simulink library "Lib_Piccolo"  (R2018b)
settings: Solver=VariableStepAuto  StartTime=0.0  StopTime=10.0  RelTol=1e-3
values from neighbouring files (symbols this model uses):
  AccelErrInt2Brakes = 0.15    [SimulationControlConfig16P.m]    (also in SimulationControlConfig16P_F0.m; SimulationControlConfig16P_F2.m; SimulationControlConfig16P_LEGACY.m; SimulationControlConfigTAILLESS.m = 0.2)
  AileronMax = 25    [SimulationControlConfig16P.m]    (also in SimulationControlConfig16P_F0.m; SimulationControlConfig16P_F2.m; SimulationControlConfig16P_LEGACY.m; SimulationControlConfigTAILLESS.m)
  AileronPower = 0.00268    [SimulationControlConfig16P.m]    (also in SimulationControlConfig16P_F0.m; SimulationControlConfig16P_F2.m; SimulationControlConfig16P_LEGACY.m; SimulationControlConfigTAILLESS.m = 0.002266)
  AileronSurfaceMax = 45    [SimulationControlConfig16P.m]    (also in SimulationControlConfig16P_F0.m; SimulationControlConfig16P_F2.m; SimulationControlConfig16P_LEGACY.m; SimulationControlConfigTAILLESS_CGAFT_F0.m = 25)
  AileronTrim = 0    [SimulationControlConfig16P.m]    (also in SimulationControlConfig16P_F0.m; SimulationControlConfig16P_F2.m; SimulationControlConfig16P_LEGACY.m; SimulationControlConfigTAILLESS.m)
  Alt = 1000 + TerrainHeight    [SimulationStateConfig.m]
  AltCruise_m = Alt * 0.3048    [SimulationControlConfig16P.m]    (also in SimulationControlConfig16P_F2.m; SimulationControlConfigTAILLESS.m = Alt/3.28084; SimulationControlConfigTAILLESS_CGAFT_F0.m = 640; SimulationControlConfigTAILLESS_CGFWD_F0.m = 640)
  AltitudeRate2PitchCmdIntegratorInit = 0.1    [SimulationControlPre.m]
  AltMax = 10000    [SimulationControlConfig16P.m]    (also in SimulationControlConfig16P_F0.m; SimulationControlConfig16P_F2.m; SimulationControlConfig16P_LEGACY.m; SimulationControlConfigTAILLESS.m)
  AltMaxAccel = 2.5    [SimulationControlConfig16P.m]    (also in SimulationControlConfig16P_F0.m = 2; SimulationControlConfig16P_F2.m = 2; SimulationControlConfig16P_LEGACY.m = 0.9; SimulationControlConfigTAILLESS.m = 2)
  AltMin = 0    [SimulationControlConfig16P.m]    (also in SimulationControlConfig16P_F0.m; SimulationControlConfig16P_F2.m; SimulationControlConfig16P_LEGACY.m; SimulationControlConfigTAILLESS.m)
  AltRateCmd2Pitch = 0.26    [SimulationControlConfig16P.m]    (also in SimulationControlConfig16P_F0.m = 0.35; SimulationControlConfig16P_F2.m = 0.35; SimulationControlConfig16P_LEGACY.m = 0.6; SimulationControlConfigTAILLESS.m = 0.9)
  AltRateError2Pitch = 0.34    [SimulationControlConfig16P.m]    (also in SimulationControlConfig16P_F0.m = 0.61; SimulationControlConfig16P_F2.m = 0.61; SimulationControlConfig16P_LEGACY.m = 0.4; SimulationControlConfigTAILLESS.m = 0.3)
  AltRateErrorInt2Pitch = 0.61    [SimulationControlConfig16P.m]    (also in SimulationControlConfig16P_F0.m = 0.28; SimulationControlConfig16P_F2.m = 0.28; SimulationControlConfig16P_LEGACY.m = 0.45; SimulationControlConfigTAILLESS.m = 0.15)
  AltRateLpfCutOff = 3    [SimulationControlConfig16P.m]    (also in SimulationControlConfig16P_F0.m; SimulationControlConfig16P_F2.m; SimulationControlConfig16P_LEGACY.m; SimulationControlConfigTAILLESS.m = 5)
  AutoNosegear2Rudder = 26    [SimulationControlConfig16P.m]    (also in SimulationControlConfig16P_F0.m; SimulationControlConfig16P_F2.m; SimulationControlConfig16P_LEGACY.m; SimulationControlConfigTAILLESS.m = 25.2)
  b = 5.54    [SimulationControlConfig16P.m]    (also in SimulationControlConfig16P_F0.m; SimulationControlConfig16P_F2.m; SimulationControlConfig16P_LEGACY.m; SimulationControlConfigTAILLESS.m = 2.37)
  Bank2AileronIntegratorInit = 0    [SimulationControlPre.m]
  BankMax_User = BankMax_User/180*pi    (= 0.610865238198)    [SimulationControlConfig16P.m]    (also in SimulationControlConfig16P_F0.m = 0.523598775598; SimulationControlConfig16P_F2.m = 0.523598775598; SimulationControlConfig16P_LEGACY.m = 0.523598775598; SimulationControlConfigTAILLESS.m = 0.558505360638)
  baseLegFlaps = 20    [SimulationControlConfig16P.m]    (also in SimulationControlConfig16P_F0.m; SimulationControlConfig16P_F2.m = 15; SimulationControlConfig16P_LEGACY.m = 0; SimulationControlConfigTAILLESS.m = 0)
  C = GeneticOpt.C    [SimulationCostFunction.m]
  c = Sw/b    (= 0.841696750903)    [SimulationControlConfig16P.m]    (also in SimulationControlConfig16P_F0.m; SimulationControlConfig16P_F2.m; SimulationControlConfig16P_LEGACY.m; SimulationControlConfigTAILLESS.m = 0.354008438819)
  cell2WheelFactorMG = 5.98    [SimulationSensorConfig16P_LEGACY.m]
  cell2WheelFactorNG = 1    [SimulationSensorConfig16P_LEGACY.m]
  cellSatMaxMG = 15000    [SimulationSensorConfig16P.m]    (also in SimulationSensorConfig16P_LEGACY.m; SimulationSensorConfigTAILLESS7P.m; SimulationSensorConfigUTAIL7P.m)
  cellSatMaxNG = 1000    [SimulationSensorConfig16P.m]    (also in SimulationSensorConfig16P_LEGACY.m; SimulationSensorConfigTAILLESS7P.m; SimulationSensorConfigUTAIL7P.m)
  cellSatMinMG = -15000    [SimulationSensorConfig16P.m]    (also in SimulationSensorConfig16P_LEGACY.m; SimulationSensorConfigTAILLESS7P.m; SimulationSensorConfigUTAIL7P.m)
  cellSatMinNG = -1000    [SimulationSensorConfig16P.m]    (also in SimulationSensorConfig16P_LEGACY.m; SimulationSensorConfigTAILLESS7P.m; SimulationSensorConfigUTAIL7P.m)
  CL_Limit = CL_Max    (= 0.54)    [SimulationControlConfig16P.m]    (also in SimulationControlConfig16P_F0.m; SimulationControlConfig16P_F2.m = 0.638; SimulationControlConfig16P_LEGACY.m; SimulationControlConfigTAILLESS.m = 0.525)
  CL_Max = 0.54    [SimulationControlConfig16P.m]    (also in SimulationControlConfig16P_F0.m; SimulationControlConfig16P_F2.m = 0.638; SimulationControlConfig16P_LEGACY.m; SimulationControlConfigTAILLESS.m = 0.525)
  CL_Max_Nom = 0.465    [SimulationControlConfig16P.m]    (also in SimulationControlConfig16P_F0.m; SimulationControlConfig16P_F2.m = 0.563; SimulationControlConfig16P_LEGACY.m; SimulationControlConfigTAILLESS.m = 0.39)
  CL_Min = 0    [SimulationControlConfig16P.m]    (also in SimulationControlConfig16P_F0.m; SimulationControlConfig16P_F2.m; SimulationControlConfig16P_LEGACY.m; SimulationControlConfigTAILLESS.m)
  ClimbMaxFraction = 0.35    [SimulationControlConfig16P.m]    (also in SimulationControlConfig16P_F0.m = 0.17; SimulationControlConfig16P_F2.m = 0.17; SimulationControlConfig16P_LEGACY.m = 0.24; SimulationControlConfigTAILLESS.m = 0.21)
  ClimboutMaxBank = 7.0    (= 7)    [SimulationControlConfig16P.m]    (also in SimulationControlConfig16P_F0.m; SimulationControlConfig16P_F2.m; SimulationControlConfig16P_LEGACY.m; SimulationControlConfigTAILLESS.m = 5)
  ClimboutTimer = 7.0    (= 7)    [SimulationControlConfig16P.m]    (also in SimulationControlConfig16P_F0.m; SimulationControlConfig16P_F2.m; SimulationControlConfig16P_LEGACY.m; SimulationControlConfigTAILLESS.m)
  dCl_per_dFlap = 0.005581818    [SimulationControlConfig16P.m]    (also in SimulationControlConfig16P_F0.m = 0; SimulationControlConfig16P_F2.m = 0.0065; SimulationControlConfig16P_LEGACY.m = 0; SimulationControlConfigTAILLESS.m = 0)
  DecelerationCmd = 3.1    [SimulationControlConfig16P.m]    (also in SimulationControlConfig16P_F0.m; SimulationControlConfig16P_F2.m; SimulationControlConfig16P_LEGACY.m; SimulationControlConfigTAILLESS.m = 0.1)
  DeRotateLogicEndTimer = abs((NoseDownLimit_Deg-1)/DeRotateRamp_Dps)    [SimulationControlConfig16P.m]    (also in SimulationControlConfig16P_F0.m; SimulationControlConfig16P_F2.m; SimulationControlConfig16P_LEGACY.m; SimulationControlConfigTAILLESS.m)
  DeRotateLogicHoldNoseUpTimer = 0.1    [SimulationControlConfig16P.m]    (also in SimulationControlConfig16P_F0.m; SimulationControlConfig16P_F2.m; SimulationControlConfig16P_LEGACY.m; SimulationControlConfigTAILLESS.m)
  DeRotateLogicTimerTimeout = 2    [SimulationControlConfig16P.m]    (also in SimulationControlConfig16P_F0.m; SimulationControlConfig16P_F2.m; SimulationControlConfig16P_LEGACY.m; SimulationControlConfigTAILLESS.m)
  DeRotateLowerCmdSaturation = 0    [SimulationControlConfig16P.m]    (also in SimulationControlConfig16P_F0.m; SimulationControlConfig16P_F2.m; SimulationControlConfig16P_LEGACY.m; SimulationControlConfigTAILLESS.m)
  DeRotateRamp_Dps = 3    [SimulationControlConfig16P.m]    (also in SimulationControlConfig16P_F0.m; SimulationControlConfig16P_F2.m; SimulationControlConfig16P_LEGACY.m; SimulationControlConfigTAILLESS.m = 8)
  DeRotateUpperCmdSaturation = 7    [SimulationControlConfig16P.m]    (also in SimulationControlConfig16P_F0.m; SimulationControlConfig16P_F2.m; SimulationControlConfig16P_LEGACY.m; SimulationControlConfigTAILLESS.m)
  DescentMaxFraction = 0.22    [SimulationControlConfig16P.m]    (also in SimulationControlConfig16P_F0.m = 0.2; SimulationControlConfig16P_F2.m = 0.2; SimulationControlConfig16P_LEGACY.m = 0.2; SimulationControlConfigTAILLESS.m = 0.17)
  DesktopSimTerrainOffset_m = 0.406    [SimulationAircraftConfig.m]
  downwindFlaps = 0    [SimulationControlConfig16P.m]    (also in SimulationControlConfig16P_F0.m; SimulationControlConfig16P_F2.m = 15; SimulationControlConfig16P_LEGACY.m; SimulationControlConfigTAILLESS.m)
  downwindSplitAil = 0    [SimulationControlConfig16P_F2.m]
  DP_init = 0.5*1.225*V_init^2    [SimulationControlConfig16P.m]    (also in SimulationControlConfig16P_F0.m; SimulationControlConfig16P_F2.m; SimulationControlConfig16P_LEGACY.m; SimulationControlConfigTAILLESS.m)
  dscNoiseMG = 1    [SimulationSensorConfig16P_LEGACY.m]
  dscNoiseNG = 0.25    [SimulationSensorConfig16P_LEGACY.m]
  DSCnumBits = 24    [SimulationSensorConfig16P.m]    (also in SimulationSensorConfig16P_LEGACY.m; SimulationSensorConfigTAILLESS7P.m; SimulationSensorConfigUTAIL7P.m)
  DSCRangeMaxMG = 15000    [SimulationSensorConfig16P.m]    (also in SimulationSensorConfig16P_LEGACY.m; SimulationSensorConfigTAILLESS7P.m; SimulationSensorConfigUTAIL7P.m)
  DSCRangeMaxNG = 1000    [SimulationSensorConfig16P.m]    (also in SimulationSensorConfig16P_LEGACY.m; SimulationSensorConfigTAILLESS7P.m; SimulationSensorConfigUTAIL7P.m)
  DSCRangeMinMG = -15000    [SimulationSensorConfig16P.m]    (also in SimulationSensorConfig16P_LEGACY.m; SimulationSensorConfigTAILLESS7P.m; SimulationSensorConfigUTAIL7P.m)
  DSCRangeMinNG = -1000    [SimulationSensorConfig16P.m]    (also in SimulationSensorConfig16P_LEGACY.m; SimulationSensorConfigTAILLESS7P.m; SimulationSensorConfigUTAIL7P.m)
  dt = DLLSim.dt    [SimulationTimeStep.m]    (also in SimulationTrim.m = 0.02)
  EarlyTouchdownThreshold = 3.0    (= 3)    [SimulationControlConfig16P.m]    (also in SimulationControlConfig16P_F0.m; SimulationControlConfig16P_F2.m; SimulationControlConfig16P_LEGACY.m; SimulationControlConfigTAILLESS.m)
  ElevatorDeflectionRate = 15    [SimulationControlConfig16P.m]    (also in SimulationControlConfig16P_F0.m; SimulationControlConfig16P_F2.m; SimulationControlConfig16P_LEGACY.m = 12; SimulationControlConfigTAILLESS.m = 5)
  ElevatorMax = 25    [SimulationControlConfig16P.m]    (also in SimulationControlConfig16P_F0.m; SimulationControlConfig16P_F2.m; SimulationControlConfig16P_LEGACY.m; SimulationControlConfigTAILLESS.m)
  ElevatorPower = -0.002209    [SimulationControlConfig16P.m]    (also in SimulationControlConfig16P_F0.m; SimulationControlConfig16P_F2.m; SimulationControlConfig16P_LEGACY.m; SimulationControlConfigTAILLESS.m = -0.002668)
  ElevatorTrim = -3.5    [SimulationControlConfig16P.m]    (also in SimulationControlConfig16P_F0.m; SimulationControlConfig16P_F2.m; SimulationControlConfig16P_LEGACY.m; SimulationControlConfigTAILLESS.m = -3)
  elevonBias = 0    [SimulationControlConfig16P.m]    (also in SimulationControlConfig16P_F0.m; SimulationControlConfig16P_F2.m; SimulationControlConfig16P_LEGACY.m; SimulationControlConfigTAILLESS.m)
  Enable_TAS_Protection = 0    [SimulationControlConfig16P.m]    (also in SimulationControlConfig16P_F0.m; SimulationControlConfig16P_F2.m; SimulationControlConfig16P_LEGACY.m; SimulationControlConfigTAILLESS.m)
  EnableCrossTrackAbort = 1    [SimulationControlConfig16P.m]    (also in SimulationControlConfigTAILLESS.m; SimulationControlConfigTAILLESS_CGAFT_F0.m; SimulationControlConfigTAILLESS_CGFWD_F0.m; SimulationControlConfigTAILLESS_CGFWD_F2.m)
  EnergyBandwidth = 0.04    [SimulationControlConfig16P.m]    (also in SimulationControlConfig16P_F0.m = 0.03; SimulationControlConfig16P_F2.m = 0.03; SimulationControlConfig16P_LEGACY.m = 0.02; SimulationControlConfigTAILLESS.m = 0.06)
  EngineLhFuelCut = 0    [SimulationAircraftConfig.m]
  EngineRhFuelCut = 0    [SimulationAircraftConfig.m]
  FastThrottleRate = 0.075    [SimulationControlConfig16P.m]    (also in SimulationControlConfig16P_F0.m = 0.05; SimulationControlConfig16P_F2.m = 0.05; SimulationControlConfig16P_LEGACY.m = 0.05; SimulationControlConfigTAILLESS.m = 0.1)
  FilterWarmUpTime = 2    [SimulationSensorConfig16P.m]    (also in SimulationSensorConfig16P_LEGACY.m; SimulationSensorConfigTAILLESS7P.m; SimulationSensorConfigUTAIL7P.m)
  finalApproachFlaps = 20    [SimulationControlConfig16P.m]    (also in SimulationControlConfig16P_F0.m; SimulationControlConfig16P_F2.m = 15; SimulationControlConfig16P_LEGACY.m = 0; SimulationControlConfigTAILLESS.m = 0)
  finalApproachSplitAil = 20    [SimulationControlConfig16P_F2.m]
  FinalDescentSlope_Deg = testPlans(testIndx).descentSlope    [SimulationControlConfig16P.m]    (also in SimulationControlConfig16P_F0.m; SimulationControlConfig16P_F2.m; SimulationControlConfig16P_LEGACY.m; SimulationControlConfigTAILLESS.m)
  flapMax = 0    [SimulationControlConfig16P.m]    (also in SimulationControlConfig16P_F0.m = 35; SimulationControlConfig16P_F2.m = 33; SimulationControlConfig16P_LEGACY.m; SimulationControlConfigTAILLESS.m)
  flapRate = 7.5    [SimulationControlConfig16P.m]    (also in SimulationControlConfig16P_F0.m; SimulationControlConfig16P_F2.m; SimulationControlConfig16P_LEGACY.m; SimulationControlConfigTAILLESS.m = 6.6)
  FlareHeight = 5    [SimulationControlConfig16P.m]    (also in SimulationControlConfig16P_F0.m; SimulationControlConfig16P_F2.m; SimulationControlConfig16P_LEGACY.m = 4.8; SimulationControlConfigTAILLESS.m = 2.75)
  FlareVerticalRate_mps = -0.4    [SimulationControlConfig16P.m]    (also in SimulationControlConfig16P_F0.m; SimulationControlConfig16P_F2.m; SimulationControlConfig16P_LEGACY.m = -0.5; SimulationControlConfigTAILLESS.m = -0.15)
  Fp_Aileron = 0.55*2*pi*RollRateLpfCutoff*dt    [SimulationControlConfig16P.m]    (also in SimulationControlConfig16P_F0.m; SimulationControlConfig16P_F2.m; SimulationControlConfig16P_LEGACY.m; SimulationControlConfigTAILLESS.m)
  Fp_Alt = 2*pi*0.55*AltBandwidth    (= 0.622035345411)    [SimulationControlConfig16P.m]    (also in SimulationControlConfig16P_F0.m; SimulationControlConfig16P_F2.m; SimulationControlConfig16P_LEGACY.m = 0.099; SimulationControlConfigTAILLESS.m = 0.207345115137)
  Fp_AltRate = 0.55*2*pi*AltRateLpfCutOff*dt    [SimulationControlConfig16P.m]    (also in SimulationControlConfig16P_F0.m; SimulationControlConfig16P_F2.m; SimulationControlConfig16P_LEGACY.m; SimulationControlConfigTAILLESS.m)
  Fp_Elevator = 0.55*2*pi*PitchRateLpfCutoff*dt    [SimulationControlConfig16P.m]    (also in SimulationControlConfig16P_F0.m; SimulationControlConfig16P_F2.m; SimulationControlConfig16P_LEGACY.m; SimulationControlConfigTAILLESS.m)
  Fp_Energy = 0.55*2*pi*EnergyBandwidth    (= 0.138230076758)    [SimulationControlConfig16P.m]    (also in SimulationControlConfig16P_F0.m = 0.103672557568; SimulationControlConfig16P_F2.m = 0.103672557568; SimulationControlConfig16P_LEGACY.m = 0.069115038379; SimulationControlConfigTAILLESS.m = 0.207345115137)
  Fp_Energy2 = 0.55*2*pi*EnergyBandwidth*dt    [SimulationControlConfig16P.m]    (also in SimulationControlConfig16P_F0.m; SimulationControlConfig16P_F2.m; SimulationControlConfig16P_LEGACY.m; SimulationControlConfigTAILLESS.m)
  Fp_Pitch = 0.55*2*pi*PitchBandwidth    (= 2.45358386245)    [SimulationControlConfig16P.m]    (also in SimulationControlConfig16P_F0.m; SimulationControlConfig16P_F2.m = 1.72787595947; SimulationControlConfig16P_LEGACY.m = 3.11017672705; SimulationControlConfigTAILLESS.m = 1.55508836353)
  Fp_Pitch_2 = 0.55*2*pi*PitchBandwidth*dt    [SimulationControlConfig16P.m]    (also in SimulationControlConfig16P_F0.m; SimulationControlConfig16P_F2.m; SimulationControlConfig16P_LEGACY.m; SimulationControlConfigTAILLESS.m)
  Fp_Roll = RollBandwidth^2    (= 1.69)    [SimulationControlConfig16P.m]    (also in SimulationControlConfig16P_F0.m = 1.44; SimulationControlConfig16P_F2.m = 1.44; SimulationControlConfig16P_LEGACY.m = 1.44; SimulationControlConfigTAILLESS.m = 1.21)
  Fp_Rudder = 0.55*2*pi*YawRateLpfCutoff*dt    [SimulationControlConfig16P.m]    (also in SimulationControlConfig16P_F0.m; SimulationControlConfig16P_F2.m; SimulationControlConfig16P_LEGACY.m; SimulationControlConfigTAILLESS.m)
  Fp_TAS = 0.55*2*pi*TASBandwidth    (= 0.103672557568)    [SimulationControlConfig16P.m]    (also in SimulationControlConfig16P_F0.m; SimulationControlConfig16P_F2.m; SimulationControlConfig16P_LEGACY.m; SimulationControlConfigTAILLESS.m = 0.172787595947)
  Fp_TAS_Filter = 2*pi*TasLpfCutoff*dt    [SimulationControlConfig16P.m]    (also in SimulationControlConfig16P_F0.m; SimulationControlConfig16P_F2.m; SimulationControlConfig16P_LEGACY.m; SimulationControlConfigTAILLESS.m)
  Fp_Turn = 0.55*2*pi*TurnErrLPFcutoff    (= 0.172787595947)    [SimulationControlConfig16P.m]    (also in SimulationControlConfig16P_F0.m = 0.0345575191895; SimulationControlConfig16P_F2.m = 0.0345575191895; SimulationControlConfig16P_LEGACY.m = 0.0345575191895; SimulationControlConfigTAILLESS.m)
  Fp_TurnDerr = 0.55*2*pi*TurnDerivativeLPFcutoff    (= 0.172787595947)    [SimulationControlConfig16P.m]    (also in SimulationControlConfig16P_F0.m = 0.0345575191895; SimulationControlConfig16P_F2.m = 0.0345575191895; SimulationControlConfig16P_LEGACY.m = 0.0345575191895; SimulationControlConfigTAILLESS.m)
  FTV = 3    [SimulationAircraftConfig.m]
  ftvStaticPositionError = 1/1.18    (= 0.847457627119)    [SimulationSensorConfig16P.m]    (also in SimulationSensorConfig16P_LEGACY.m; SimulationSensorConfigTAILLESS7P.m = 1; SimulationSensorConfigUTAIL7P.m = 1)
  g = 9.81    [SimulationStateConfig.m]
  goAroundSplitAil = 0    [SimulationControlConfig16P_F2.m]
  GustSpd_Kts = testPlans(testIndx).gustSpd    [SimulationStateConfig.m]
  GustTriggerVal = testPlans(testIndx).gustTriggerVal    [SimulationStateConfig.m]
  HeadingErr2TurnRate = 0.5    [SimulationControlConfig16P.m]    (also in SimulationControlConfig16P_F0.m; SimulationControlConfig16P_F2.m; SimulationControlConfig16P_LEGACY.m; SimulationControlConfigTAILLESS.m)
  HeadingErrDer2TurnRate = 0.3    [SimulationControlConfig16P.m]    (also in SimulationControlConfig16P_F0.m; SimulationControlConfig16P_F2.m; SimulationControlConfig16P_LEGACY.m; SimulationControlConfigTAILLESS.m)
  IASbounce = IASstall*0.8    [SimulationControlPre.m]
  IAScruiseCMD = sqrt(2*m*9.81/(1.225*Sw*CL_cruise))    [SimulationControlConfig16P.m]    (also in SimulationControlConfig16P_F0.m; SimulationControlConfig16P_F2.m; SimulationControlConfig16P_LEGACY.m; SimulationControlConfigTAILLESS.m)
  IASfinalCMD = 1.12 * IASmin    [SimulationControlConfig16P.m]    (also in SimulationControlConfig16P_F0.m = 1.14 * IASmin; SimulationControlConfig16P_F2.m = 1.10 * IASmin; SimulationControlConfig16P_LEGACY.m = 1.10 * IASmin; SimulationControlConfigTAILLESS.m = 1.14 * IASmin)
  IASflareCMD = IASstall    [SimulationControlConfig16P.m]    (also in SimulationControlConfig16P_F0.m; SimulationControlConfig16P_F2.m; SimulationControlConfig16P_LEGACY.m; SimulationControlConfigTAILLESS.m)
  IASmax = 64    [SimulationControlConfig16P.m]    (also in SimulationControlConfig16P_F0.m = 46; SimulationControlConfig16P_F2.m = 52; SimulationControlConfig16P_LEGACY.m = 46; SimulationControlConfigTAILLESS.m = 38.9)
  IASmin = sqrt(2*m*9.81/(1.225*Sw*0.9*CL_Max_Nom))    [SimulationControlConfig16P.m]    (also in SimulationControlConfig16P_F0.m; SimulationControlConfig16P_F2.m; SimulationControlConfig16P_LEGACY.m; SimulationControlConfigTAILLESS.m)
  IASshortCMD = IASstall    [SimulationControlConfig16P.m]    (also in SimulationControlConfig16P_F0.m; SimulationControlConfig16P_F2.m; SimulationControlConfig16P_LEGACY.m; SimulationControlConfigTAILLESS.m)
  IASstall = sqrt(2*m*9.81/(1.225*Sw*CL_Max))    [SimulationControlConfig16P.m]    (also in SimulationControlConfig16P_F0.m; SimulationControlConfig16P_F2.m; SimulationControlConfig16P_LEGACY.m; SimulationControlConfigTAILLESS.m)
  inFlight = 1    [SimulationControlConfig16P.m]    (also in SimulationControlConfigTAILLESS.m; SimulationControlConfigTAILLESS_CGAFT_F0.m; SimulationControlConfigTAILLESS_CGFWD_F0.m; SimulationControlConfigTAILLESS_CGFWD_F2.m)
  JetCatOffset = 5    [SimulationControlConfig16P.m]    (also in SimulationControlConfig16P_F0.m; SimulationControlConfig16P_F2.m; SimulationControlConfig16P_LEGACY.m)
  LaunchRollingElevator = -1.5    [SimulationControlConfig16P.m]    (also in SimulationControlConfig16P_F0.m; SimulationControlConfig16P_F2.m = 1.25; SimulationControlConfig16P_LEGACY.m; SimulationControlConfigTAILLESS.m = 1)
  ldg_NosegearMax = 10    [SimulationControlConfig16P.m]    (also in SimulationControlConfig16P_F0.m; SimulationControlConfig16P_F2.m; SimulationControlConfig16P_LEGACY.m; SimulationControlConfigTAILLESS.m)
  ldg_TrackVyErrInt2Nosegear = 0.1250    (= 0.125)    [SimulationControlConfig16P.m]    (also in SimulationControlConfig16P_F0.m; SimulationControlConfig16P_F2.m; SimulationControlConfig16P_LEGACY.m; SimulationControlConfigTAILLESS.m = 0.00714285714286)
  ldg_TrackVyErrPro2Nosegear = 0.35    [SimulationControlConfig16P.m]    (also in SimulationControlConfig16P_F0.m; SimulationControlConfig16P_F2.m; SimulationControlConfig16P_LEGACY.m; SimulationControlConfigTAILLESS.m = 0.0546666666667)
  ldg_TrackY2Vy = 0.07    [SimulationControlConfig16P.m]    (also in SimulationControlConfig16P_F0.m; SimulationControlConfig16P_F2.m; SimulationControlConfig16P_LEGACY.m; SimulationControlConfigTAILLESS.m = 0.17)
  ldg_Vy2NosegearScalingPower = 1.075    [SimulationControlConfig16P.m]    (also in SimulationControlConfig16P_F0.m; SimulationControlConfig16P_F2.m; SimulationControlConfig16P_LEGACY.m; SimulationControlConfigTAILLESS.m = 0.6)
  ldg_Y2VyScalingPower = 0.175    [SimulationControlConfig16P.m]    (also in SimulationControlConfig16P_F0.m; SimulationControlConfig16P_F2.m; SimulationControlConfig16P_LEGACY.m; SimulationControlConfigTAILLESS.m = 0)
  ldg_YawRate2Nosegear = 0.175    [SimulationControlConfig16P.m]    (also in SimulationControlConfig16P_F0.m; SimulationControlConfig16P_F2.m; SimulationControlConfig16P_LEGACY.m; SimulationControlConfigTAILLESS.m = 0.065)
  LiftSlope = 0.064285    [SimulationControlConfig16P.m]    (also in SimulationControlConfig16P_F0.m; SimulationControlConfig16P_F2.m; SimulationControlConfig16P_LEGACY.m; SimulationControlConfigTAILLESS.m = 0.058631)
  LPFaileronInit = 0    [SimulationControlPre.m]
  LPFclestInit = 0    [SimulationControlPre.m]
  LPFenergyFFInit = 0    [SimulationControlPre.m]
  ... (+122 more)
undefined symbols (not defined in the file or in its folder): abortFlag, alphaHPF, apmDelay, BRWNOUT, CRAWOR, CRAWUR, DiscIntNeverNeededParam, DLLSim, DLLSimStep, ECOMOR, ECOMUR, Fp_Tas, GustTrigger_HeightAgl_m, IPSTAT, LCINTEG, Ldg_Persist_Time, LOWER_FLAGS, MSG_ENABLE, NoiseStd, OLDVAL, OVERRIDE_ENABLE, OVERRIDE_VALUE, REBOOT, reversionEnable, revIASMax, revIASMin, revPitchMax, revPitchMin, revPitchRateMax, revRollMax, revRollRateMax, SAMPLE, SCALON, SensorModel, sigbuilder_block, Sim_Vx, Sim_Vy, Sim_Vz, Sim_Xpos, Sim_Ypos, Sim_Zpos, SYSOR, SYSUR, TARE, TEMPOR, TEMPUR, testIndx, testPlan, testPlans, Trim_piccoloInCmd, Trim_REFSI_FD_IN_nmodeCgShifterCmd_Flag, Trim_REFSI_FD_IN_nmodeCgShifterCmd_Ft, Trim_REFSI_FD_IN_nmodeCgShifterCmdType, Trim_REFSI_FD_IN_nmodeCgShifterNRCActive, Trim_REFSI_FD_IN_nmodeFlapLhIBCmd_Deg, Trim_REFSI_FD_IN_nmodeFlapLhOBCmd_Deg, Trim_REFSI_FD_IN_nmodeFlapRhIBCmd_Deg, Trim_REFSI_FD_IN_nmodeFlapRhOBCmd_Deg, Trim_REFSI_FD_IN_nmodeSlatLhCmd_Deg ... (+11)
libraries: simulink x1237, $bdroot x179, aerolibconvert2 x63, dspswit3 x25, aerolibatmos2 x5, simulink_extras x4, dsparch4 x2, Lib_Piccolo_Alt x2, eeGeneralControl x1, dspindex x1
(part 6 of 74)

== system Lib_Piccolo/Throttle Control (Alt Mode) ==
  note: !!!!!!!There is a missing feedforward based on "load factor". This relates to current turn
  hdotCmd : Inport
  TAScmd : Inport  Port=2
  Feedback Bus : Inport  Port=3
  " " : Constant  Value=ThrottleTrim
  " TLASaturation " : Saturate  UpperLimit=ThrottleMax  LowerLimit=ThrottleMin  LinearizeAsGain=off
  "1/ MaxEnginePower " : Gain  Gain=1/MaxEnginePower
  "1/ MaxEnginePower " : Gain  Gain=1/MaxEnginePower
  1st Order Reference Model : Subsystem
  Bus Selector : BusSelector  OutputSignals=V_mps,Vdot_mps2,apMode
  Compare To Constant3 : simulink/Logic and Bit Operations/Compare To Constant  relop=>=  const=11  OutDataTypeStr=boolean
  Constant2 : Constant  Value=0
  Constant3 : Constant  Value=ThrottleRateMax
  Constant4 : Constant  Value=ThrottleControlAltitudeModeIntegratorInit
  Constant5 : Constant  Value=100
  Discrete-Time Integrator1 : DiscreteIntegrator  IntegratorMethod=Integration: Backward Euler  ExternalReset=level  InitialConditionSource=external  SampleTime=-1  LimitOutput=on  UpperSaturationLimit=ThrottleMax-ThrottleTrim  LowerSaturationLimit=ThrottleMin-ThrottleTrim  ICPrevOutput=DiscIntNeverNeededParam  ICPrevScaledInput=DiscIntNeverNeededParam
  Divide : Product  Inputs=**
  EngineKill : Constant  Value=0
  Filter and Throttle Cut : Subsystem
  Flare Throttle Modifications 2 : Subsystem
  Gain : Gain  Gain=m/2
  Gain1 : Gain  Gain=m
  Gain2 : Gain  Gain=m*g
  Gain3 : Gain  Gain=m/2
  Gain4 : Gain  Gain=-1
  KI_Power : Gain  Gain=PowerErrorInt2Throttle
  Kp_Power : Gain  Gain=PowerError2Throttle
  LPF Energy Alpha : Subsystem
  NOT1 : Logic  Operator=NOT  IconShape=distinctive  AllPortsSameDT=off  OutDataTypeStr=boolean
  O/L Throttle Ramp : Subsystem
  Rate Limiter Dynamic : simulink/Discontinuities/Rate Limiter Dynamic
      settings: SourceProductName=Simulink
  Reset Conditions : Subsystem
  Speed Flags : Subsystem
  Square : Math  Operator=square  SaturateOnIntegerOverflow=on
  Square1 : Math  Operator=square  SaturateOnIntegerOverflow=on
  Sum : Sum  Inputs=|+-
  Sum1 : Sum  Inputs=|++
  Sum3 : Sum  Inputs=|++
  Sum4 : Sum  Inputs=+++
  Sum5 : Sum  Inputs=|+-
  Switch : Switch  Criteria=u2 > Threshold  Threshold=0.5
  Switch1 : Switch  Criteria=u2 > Threshold  Threshold=5
  Switch2 : Switch  Criteria=u2 > Threshold  Threshold=0.5
  Switch3 : Switch  Criteria=u2 > Threshold  Threshold=3
  Switch9 : Switch  Criteria=u2 > Threshold
  ThrottlePredictionTrust : Gain  Gain=ThrottlePredictionTrust
  Throttle (Alt TEC) : Outport
  tag scope: Flag_Overspeed=global, Flag_Underspeed=global, Sim_TASError=global, Throttle_Post_Slew=global, Throttle_Pre_Slew=global
  wires:
  TAScmd/1 -> Sum5/1, Switch9/3
  Square/1 -> Gain/1
  Divide/1 -> Gain1/1
  Sum/1 -> "1/ MaxEnginePower "/1
  "1/ MaxEnginePower "/1 -> Kp_Power/1, KI_Power/1  "Sim.Power Error"
  Sum1/1 -> ThrottlePredictionTrust/1
  "1/ MaxEnginePower "/1 -> Sum4/1  "Feedforward_Power"
  1st Order Reference Model/1(Rf) -> Sum1/2, Sum/1
  Gain/1 -> 1st Order Reference Model/1(Pcmd)
  Square1/1 -> Gain3/1
  Bus Selector/2 -> Divide/2  "<Vdot_mps2>"
  Sum5/1 -> [Sim_TASError]  "Sim_TASError"
  LPF Energy Alpha/1(Output) -> Gain2/1
  hdotCmd/1 -> LPF Energy Alpha/1(Input)
  KI_Power/1 -> Discrete-Time Integrator1/1
  Sum4/1 -> Sum3/1  "PI"
  Constant4/1 -> Switch1/1
  Discrete-Time Integrator1/1 -> Sum4/3  "KI_Power"
  Bus Selector/3 -> Reset Conditions/1(AP Mode), Switch3/2, Flare Throttle Modifications 2/3(AP Mode (0 - 12)), Filter and Throttle Cut/3(apMode), Switch1/2, Compare To Constant3/1  "<apMode>"
  ThrottlePredictionTrust/1 -> "1/ MaxEnginePower "/1
  Gain2/1 -> Sum1/1
  Gain3/1 -> 1st Order Reference Model/2(Pact)
  Kp_Power/1 -> Sum4/2  "Kp_Power"
  Switch1/1 -> Discrete-Time Integrator1/3
  Constant2/1 -> Switch9/1
  Gain1/1 -> Sum/2
  Switch9/1 -> Square/1
  Rate Limiter Dynamic/1 -> " TLASaturation "/1
  Sum3/1 -> Switch/1
  Bus Selector/1 -> Sum5/2, Square1/1, 1st Order Reference Model/3("V "), Divide/1  "<V_mps>"
  Compare To Constant3/1 -> Switch9/2
  [ApGlobal] -> Switch/2, Switch2/2, NOT1/1
  NOT1/1 -> Filter and Throttle Cut/2(Reset LPF)
  " TLASaturation "/1 -> Filter and Throttle Cut/1(Throttle In)
  Constant3/1 -> Switch2/1
  Switch2/1 -> Gain4/1, Rate Limiter Dynamic/1
  Gain4/1 -> Rate Limiter Dynamic/3
  Constant5/1 -> Switch2/3
  [pilotThr] -> Switch/3
  Switch/1 -> Rate Limiter Dynamic/2
  " "/1 -> Sum3/2
  Speed Flags/1(Flag_Underspeed) -> [Flag_Underspeed]
  Speed Flags/2(Flag_Overspeed) -> [Flag_Overspeed]
  Filter and Throttle Cut/1(Throttle Out) -> [Throttle_Pre_Slew], Flare Throttle Modifications 2/1(Throttle In (0 - 100%))
  Flare Throttle Modifications 2/1(Throttle Out) -> [Throttle_Post_Slew], Switch3/1
  [PicElevatorOut] -> Flare Throttle Modifications 2/2(Piccolo Elevator In (deg.))
  O/L Throttle Ramp/1(Sim.LaunchThrottleCmd) -> Switch3/3, Switch1/3, Filter and Throttle Cut/4(Throttle Ramp In)
  Feedback Bus/1 -> Bus Selector/1, Speed Flags/1(Feedback Bus), O/L Throttle Ramp/1(Feedback Bus)
  Switch3/1 -> Throttle (Alt TEC)/1
  [startTaxi] -> O/L Throttle Ramp/2(startFlag)
  Reset Conditions/1(Reset) -> Discrete-Time Integrator1/2
  [TakeoffAbortFlag] -> Flare Throttle Modifications 2/5(RTOActive In)
  [ApGlobal] -> Flare Throttle Modifications 2/4(ApGlobal In)
  EngineKill/1 -> Flare Throttle Modifications 2/6(EngineKill In)

== system Lib_Piccolo/VRate Reference Selection ==
  note: Allows Rate Limiter to track current value during AP-off where rates can be arbitrary.
      | Should investigate using a resettable rate limiter to avoid hardcoded value (gross!)
  VRateCmd (Alt) : Inport
  LonMode : Inport  Port=2
  VRateCmd (TAS) : Inport  Port=3
  AND : Logic  IconShape=distinctive  AllPortsSameDT=off  OutDataTypeStr=boolean
  AND1 : Logic  IconShape=distinctive  AllPortsSameDT=off  OutDataTypeStr=boolean
  AND2 : Logic  IconShape=distinctive  AllPortsSameDT=off  OutDataTypeStr=boolean
  Alt Max Accel Rate Limit : Subsystem
  Compare To Constant : simulink/Logic and Bit Operations/Compare To Constant  relop===  const=1  OutDataTypeStr=boolean
  Compare To Constant1 : simulink/Logic and Bit Operations/Compare To Constant  relop=<  const=10  OutDataTypeStr=boolean
  Compare To Constant2 : simulink/Logic and Bit Operations/Compare To Constant  relop=>  const=0  OutDataTypeStr=boolean
  Constant : Constant  Value=Enable_TAS_Protection
  Constant4 : Constant  Value=AltMaxAccel
  Constant5 : Constant  Value=100
  Gain : Gain  Gain=-1
  OR : Logic  Operator=OR  IconShape=distinctive  AllPortsSameDT=off  OutDataTypeStr=boolean
  OR1 : Logic  Operator=OR  IconShape=distinctive  AllPortsSameDT=off  OutDataTypeStr=boolean
  Switch : Switch  Criteria=u2 > Threshold
  Switch2 : Switch  Criteria=u2 > Threshold  Threshold=0.5
  VRateCmd : Outport
  tag scope: Flag_TAS_Priority=global
  wires:
  Switch/1 -> Alt Max Accel Rate Limit/2(u)
  Alt Max Accel Rate Limit/1(Y) -> VRateCmd/1  "Sim.VRateCmd"
  Compare To Constant/1 -> OR/1
  LonMode/1 -> Compare To Constant/1
  VRateCmd (Alt)/1 -> Switch/3
  VRateCmd (TAS)/1 -> Switch/1
  AND/1 -> AND1/1, Switch/2  "Flag_TAS_Priority"
  Constant5/1 -> Switch2/3
  Switch2/1 -> Alt Max Accel Rate Limit/1(up), Gain/1  "altAccelLimit"
  [ApGlobal] -> Switch2/2
  Constant4/1 -> Switch2/1
  Gain/1 -> Alt Max Accel Rate Limit/3(lo)
  [ApGlobal] -> AND/1
  OR/1 -> AND/2
  AND1/1 -> [Flag_TAS_Priority]
  Compare To Constant1/1 -> AND1/2
  [Pic_AP_Mode] -> Compare To Constant1/1
  Compare To Constant2/1 -> AND2/2
  Constant/1 -> Compare To Constant2/1
  [Flag_Underspeed] -> OR1/1
  [Flag_Overspeed] -> OR1/2
  OR1/1 -> AND2/1
  AND2/1 -> OR/2

== system Lib_Piccolo/WOW Archive Container ==
  note: 15 - Landing logic matched to LOAD14, differs in takeoff:
      | - Ability to use Piccolo mode changes as analog for airspeed to drive weight-off-wheels signal
  note: 14 - Logic derived from LOAD2, with key changes:
      | - Saturation on inputs to filter to prevent 'wind-up'
  note: 17 - Landing logic matched to LOAD16, differs in takeoff:
      | - Ability to use Piccolo mode changes as analog for airspeed to drive weight-off-wheels signal
  Load Cell WoW Model 10 : Subsystem  VariantControl="SensorModel.WOW.Cell.Variant==\"LOAD10\""
  Load Cell WoW Model 10_OLD : Subsystem  VariantControl="SensorModel.WOW.Cell.Variant==\"LOAD10_OLD\""
  Load Cell WoW Model 11 : Subsystem  VariantControl="SensorModel.WOW.Cell.Variant==\"LOAD11\""
  Load Cell WoW Model 11_OLD : Subsystem  VariantControl="SensorModel.WOW.Cell.Variant==\"LOAD11_OLD\""
  Load Cell WoW Model 12 : Subsystem  VariantControl="SensorModel.WOW.Cell.Variant==\"LOAD12\""
  Load Cell WoW Model 14 : Subsystem  VariantControl="SensorModel.WOW.Cell.Variant==\"LOAD14\""
  Load Cell WoW Model 15 : Subsystem  VariantControl="SensorModel.WOW.Cell.Variant==\"LOAD15\""
  Load Cell WoW Model 17 : Subsystem  VariantControl="SensorModel.WOW.Cell.Variant==\"LOAD17\""
  Load Cell WoW Model 2 : Subsystem  VariantControl="SensorModel.WOW.Cell.Variant==\"LOAD2\""
  Load Cell WoW Model 3 - LiftOff Delay : Subsystem  VariantControl="SensorModel.WOW.Cell.Variant==\"LOAD3\""  mask{Ldg_Persist_Time=SensorModel.WOW.Cell.persistanceTime_s, Ldg_Latch_Time_P=SensorModel.WOW.Cell.longLatchTime_s, Ldg_Latch_Time_S=SensorModel.WOW.Cell.shortLatchTime_s, Ldg_Load_Thresh_Upper=SensorModel.WOW.Cell.loadThresholdUpper_N, Ldg_Load_Thresh_Lower=SensorModel.WOW.Cell.loadThresholdLower_N, TO_Persist_Time=SensorModel.WOW.Cell.TO_persistanceTime_s, TO_Latch_Time=SensorModel.WOW.Cell.TO_latchTime_s, TO_Load_Thresh=SensorModel.WOW.Cell.TO_loadThreshold_N, DSCnumBits=24, numBits=16, satMaxMG=15000, satMinMG=-300, dscNoiseMG=1, DSCRangeMaxMG=15000, DSCRangeMinMG=-15000, satMaxNG=1000, satMinNG=-250, dscNoiseNG=0.25, DSCRangeMaxNG=1000, DSCRangeMinNG=-1000, cellSatMaxMG=15000, cellSatMinMG=-15000, cell2WheelFactorMG=5.98, cellSatMaxNG=1000, cellSatMinNG=-1000, cell2WheelFactorNG=1}
      mask prompts: Ldg_Persist_Time "Landing Persistance Time [s]"; Ldg_Latch_Time_P "Primary Landing Latch Time [s]"; Ldg_Latch_Time_S "Secondary Landing Latch Time [s]"; Ldg_Load_Thresh_Upper "Landing Load Threshold Upper [N]"; Ldg_Load_Thresh_Lower "Landing Load Threshold Lower [N]"; TO_Persist_Time "Take Off Persistance Time [s]"; TO_Latch_Time "Take Off Latch Time [s]"; TO_Load_Thresh "Take Off Load Threshold  [N]"; DSCnumBits "DSC Encoded Resolution [num bits]"; numBits "CANBridge Encoded Resolution [num bits]"; satMaxMG "Main Gear CANBridge Saturation Max [N]"; satMinMG "Main Gear CANBridge Saturation Min [N]"; dscNoiseMG "Main Gear DSC Noise Level pk-pk [N]"; DSCRangeMaxMG "Main Gear DSC Range Max [N]"; DSCRangeMinMG "Main Gear DSC Range Min [N]"; satMaxNG "Nose Gear CANBridge Saturation Max [N]"; satMinNG "Nose Gear CANBridge Saturation Min [N]"; dscNoiseNG "Nose Gear DSC Noise Level pk-pk [N]"; DSCRangeMaxNG "Nose Gear DSC Range Max [N]"; DSCRangeMinNG "Nose Gear DSC Range Min [N]"; cellSatMaxMG "Main Gear Cell Saturation Max [N]"; cellSatMinMG "Main Gear Cell Saturation Min [N]"; cell2WheelFactorMG "Main Gear Cell to Wheel Load Scale Factor"; cellSatMaxNG "Nose Gear Cell Saturation Max [N]"; cellSatMinNG "Nose Gear Cell Saturation Min [N]"; cell2WheelFactorNG "Nose Gear Cell to Wheel Load Scale Factor"
      mask DialogControl DescGroupVar Prompt: Full model of load-cell based weight-on-wheels system.
      mask DialogControl LogicGroupVar Prompt: Logic Configuration
      mask DialogControl DataGroupVar Prompt: Data Acquisition
      mask DialogControl Container5 Prompt: MG
      mask DialogControl Container6 Prompt: NG
      mask DialogControl ParamGroupVar Prompt: Physical Parameters
      mask DialogControl Container8 Prompt: MG
      mask DialogControl Container9 Prompt: NG
  Load Cell WoW Model 4 - LiftOff Delay variation 2 : Subsystem  VariantControl="SensorModel.WOW.Cell.Variant==\"LOAD4\""  mask{Ldg_Persist_Time=SensorModel.WOW.Cell.persistanceTime_s, Ldg_Latch_Time_P=SensorModel.WOW.Cell.longLatchTime_s, Ldg_Latch_Time_S=SensorModel.WOW.Cell.shortLatchTime_s, Ldg_Load_Thresh_Upper=SensorModel.WOW.Cell.loadThresholdUpper_N, Ldg_Load_Thresh_Lower=SensorModel.WOW.Cell.loadThresholdLower_N, TO_Persist_Time=SensorModel.WOW.Cell.TO_persistanceTime_s, TO_Latch_Time=SensorModel.WOW.Cell.TO_latchTime_s, TO_Load_Thresh=SensorModel.WOW.Cell.TO_loadThreshold_N, DSCnumBits=24, numBits=16, satMaxMG=15000, satMinMG=-300, dscNoiseMG=1, DSCRangeMaxMG=15000, DSCRangeMinMG=-15000, satMaxNG=1000, satMinNG=-250, dscNoiseNG=0.25, DSCRangeMaxNG=1000, DSCRangeMinNG=-1000, cellSatMaxMG=15000, cellSatMinMG=-15000, cell2WheelFactorMG=5.98, cellSatMaxNG=1000, cellSatMinNG=-1000, cell2WheelFactorNG=1}
      mask prompts: Ldg_Persist_Time "Landing Persistance Time [s]"; Ldg_Latch_Time_P "Primary Landing Latch Time [s]"; Ldg_Latch_Time_S "Secondary Landing Latch Time [s]"; Ldg_Load_Thresh_Upper "Landing Load Threshold Upper [N]"; Ldg_Load_Thresh_Lower "Landing Load Threshold Lower [N]"; TO_Persist_Time "Take Off Persistance Time [s]"; TO_Latch_Time "Take Off Latch Time [s]"; TO_Load_Thresh "Take Off Load Threshold  [N]"; DSCnumBits "DSC Encoded Resolution [num bits]"; numBits "CANBridge Encoded Resolution [num bits]"; satMaxMG "Main Gear CANBridge Saturation Max [N]"; satMinMG "Main Gear CANBridge Saturation Min [N]"; dscNoiseMG "Main Gear DSC Noise Level pk-pk [N]"; DSCRangeMaxMG "Main Gear DSC Range Max [N]"; DSCRangeMinMG "Main Gear DSC Range Min [N]"; satMaxNG "Nose Gear CANBridge Saturation Max [N]"; satMinNG "Nose Gear CANBridge Saturation Min [N]"; dscNoiseNG "Nose Gear DSC Noise Level pk-pk [N]"; DSCRangeMaxNG "Nose Gear DSC Range Max [N]"; DSCRangeMinNG "Nose Gear DSC Range Min [N]"; cellSatMaxMG "Main Gear Cell Saturation Max [N]"; cellSatMinMG "Main Gear Cell Saturation Min [N]"; cell2WheelFactorMG "Main Gear Cell to Wheel Load Scale Factor"; cellSatMaxNG "Nose Gear Cell Saturation Max [N]"; cellSatMinNG "Nose Gear Cell Saturation Min [N]"; cell2WheelFactorNG "Nose Gear Cell to Wheel Load Scale Factor"
      mask DialogControl DescGroupVar Prompt: Full model of load-cell based weight-on-wheels system.
      mask DialogControl LogicGroupVar Prompt: Logic Configuration
      mask DialogControl DataGroupVar Prompt: Data Acquisition
      mask DialogControl Container5 Prompt: MG
      mask DialogControl Container6 Prompt: NG
      mask DialogControl ParamGroupVar Prompt: Physical Parameters
      mask DialogControl Container8 Prompt: MG
      mask DialogControl Container9 Prompt: NG
  Load Cell WoW Model 5 - Dynamic Timing : Subsystem  VariantControl="SensorModel.WOW.Cell.Variant==\"LOAD5\""  mask{Ldg_Persist_Time=SensorModel.WOW.Cell.persistanceTime_s, Ldg_Latch_Time_P=SensorModel.WOW.Cell.longLatchTime_s, Ldg_Latch_Time_S=SensorModel.WOW.Cell.shortLatchTime_s, Ldg_Load_Thresh_Upper=SensorModel.WOW.Cell.loadThresholdUpper_N, Ldg_Load_Thresh_Lower=SensorModel.WOW.Cell.loadThresholdLower_N, TO_Persist_Time=SensorModel.WOW.Cell.TO_persistanceTime_s, TO_Latch_Time=SensorModel.WOW.Cell.TO_latchTime_s, TO_Load_Thresh=SensorModel.WOW.Cell.TO_loadThreshold_N, DSCnumBits=24, numBits=16, satMaxMG=15000, satMinMG=-300, dscNoiseMG=1, DSCRangeMaxMG=15000, DSCRangeMinMG=-15000, satMaxNG=1000, satMinNG=-250, dscNoiseNG=0.25, DSCRangeMaxNG=1000, DSCRangeMinNG=-1000, cellSatMaxMG=15000, cellSatMinMG=-15000, cell2WheelFactorMG=5.98, cellSatMaxNG=1000, cellSatMinNG=-1000, cell2WheelFactorNG=1}
      mask prompts: Ldg_Persist_Time "Landing Persistance Time [s]"; Ldg_Latch_Time_P "Primary Landing Latch Time [s]"; Ldg_Latch_Time_S "Secondary Landing Latch Time [s]"; Ldg_Load_Thresh_Upper "Landing Load Threshold Upper [N]"; Ldg_Load_Thresh_Lower "Landing Load Threshold Lower [N]"; TO_Persist_Time "Take Off Persistance Time [s]"; TO_Latch_Time "Take Off Latch Time [s]"; TO_Load_Thresh "Take Off Load Threshold  [N]"; DSCnumBits "DSC Encoded Resolution [num bits]"; numBits "CANBridge Encoded Resolution [num bits]"; satMaxMG "Main Gear CANBridge Saturation Max [N]"; satMinMG "Main Gear CANBridge Saturation Min [N]"; dscNoiseMG "Main Gear DSC Noise Level pk-pk [N]"; DSCRangeMaxMG "Main Gear DSC Range Max [N]"; DSCRangeMinMG "Main Gear DSC Range Min [N]"; satMaxNG "Nose Gear CANBridge Saturation Max [N]"; satMinNG "Nose Gear CANBridge Saturation Min [N]"; dscNoiseNG "Nose Gear DSC Noise Level pk-pk [N]"; DSCRangeMaxNG "Nose Gear DSC Range Max [N]"; DSCRangeMinNG "Nose Gear DSC Range Min [N]"; cellSatMaxMG "Main Gear Cell Saturation Max [N]"; cellSatMinMG "Main Gear Cell Saturation Min [N]"; cell2WheelFactorMG "Main Gear Cell to Wheel Load Scale Factor"; cellSatMaxNG "Nose Gear Cell Saturation Max [N]"; cellSatMinNG "Nose Gear Cell Saturation Min [N]"; cell2WheelFactorNG "Nose Gear Cell to Wheel Load Scale Factor"
      mask DialogControl DescGroupVar Prompt: Full model of load-cell based weight-on-wheels system.
      mask DialogControl LogicGroupVar Prompt: Logic Configuration
      mask DialogControl DataGroupVar Prompt: Data Acquisition
      mask DialogControl Container5 Prompt: MG
      mask DialogControl Container6 Prompt: NG
      mask DialogControl ParamGroupVar Prompt: Physical Parameters
      mask DialogControl Container8 Prompt: MG
      mask DialogControl Container9 Prompt: NG
  Load Cell WoW Model 6 - LiftOff Delay variation 3 : Subsystem  VariantControl="SensorModel.WOW.Cell.Variant==\"LOAD6\""  mask{Ldg_Persist_Time=SensorModel.WOW.Cell.persistanceTime_s, Ldg_Latch_Time_P=SensorModel.WOW.Cell.longLatchTime_s, Ldg_Latch_Time_S=SensorModel.WOW.Cell.shortLatchTime_s, Ldg_Load_Thresh_Upper=SensorModel.WOW.Cell.loadThresholdUpper_N, Ldg_Load_Thresh_Lower=SensorModel.WOW.Cell.loadThresholdLower_N, TO_Persist_Time=SensorModel.WOW.Cell.TO_persistanceTime_s, TO_Latch_Time=SensorModel.WOW.Cell.TO_latchTime_s, TO_Load_Thresh=SensorModel.WOW.Cell.TO_loadThreshold_N, DSCnumBits=24, numBits=16, satMaxMG=15000, satMinMG=-300, dscNoiseMG=1, DSCRangeMaxMG=15000, DSCRangeMinMG=-15000, satMaxNG=1000, satMinNG=-250, dscNoiseNG=0.25, DSCRangeMaxNG=1000, DSCRangeMinNG=-1000, cellSatMaxMG=15000, cellSatMinMG=-15000, cell2WheelFactorMG=5.98, cellSatMaxNG=1000, cellSatMinNG=-1000, cell2WheelFactorNG=1}
      mask prompts: Ldg_Persist_Time "Landing Persistance Time [s]"; Ldg_Latch_Time_P "Primary Landing Latch Time [s]"; Ldg_Latch_Time_S "Secondary Landing Latch Time [s]"; Ldg_Load_Thresh_Upper "Landing Load Threshold Upper [N]"; Ldg_Load_Thresh_Lower "Landing Load Threshold Lower [N]"; TO_Persist_Time "Take Off Persistance Time [s]"; TO_Latch_Time "Take Off Latch Time [s]"; TO_Load_Thresh "Take Off Load Threshold  [N]"; DSCnumBits "DSC Encoded Resolution [num bits]"; numBits "CANBridge Encoded Resolution [num bits]"; satMaxMG "Main Gear CANBridge Saturation Max [N]"; satMinMG "Main Gear CANBridge Saturation Min [N]"; dscNoiseMG "Main Gear DSC Noise Level pk-pk [N]"; DSCRangeMaxMG "Main Gear DSC Range Max [N]"; DSCRangeMinMG "Main Gear DSC Range Min [N]"; satMaxNG "Nose Gear CANBridge Saturation Max [N]"; satMinNG "Nose Gear CANBridge Saturation Min [N]"; dscNoiseNG "Nose Gear DSC Noise Level pk-pk [N]"; DSCRangeMaxNG "Nose Gear DSC Range Max [N]"; DSCRangeMinNG "Nose Gear DSC Range Min [N]"; cellSatMaxMG "Main Gear Cell Saturation Max [N]"; cellSatMinMG "Main Gear Cell Saturation Min [N]"; cell2WheelFactorMG "Main Gear Cell to Wheel Load Scale Factor"; cellSatMaxNG "Nose Gear Cell Saturation Max [N]"; cellSatMinNG "Nose Gear Cell Saturation Min [N]"; cell2WheelFactorNG "Nose Gear Cell to Wheel Load Scale Factor"
      mask DialogControl DescGroupVar Prompt: Full model of load-cell based weight-on-wheels system.
      mask DialogControl LogicGroupVar Prompt: Logic Configuration
      mask DialogControl DataGroupVar Prompt: Data Acquisition
      mask DialogControl Container5 Prompt: MG
      mask DialogControl Container6 Prompt: NG
      mask DialogControl ParamGroupVar Prompt: Physical Parameters
      mask DialogControl Container8 Prompt: MG
      mask DialogControl Container9 Prompt: NG
  Load Cell WoW Model 7 - LiftOff Delay variation 4 : Subsystem  VariantControl="SensorModel.WOW.Cell.Variant==\"LOAD7\""  mask{Ldg_Persist_Time=SensorModel.WOW.Cell.persistanceTime_s, Ldg_Latch_Time_P=SensorModel.WOW.Cell.longLatchTime_s, Ldg_Latch_Time_S=SensorModel.WOW.Cell.shortLatchTime_s, Ldg_Load_Thresh_Upper=SensorModel.WOW.Cell.loadThresholdUpper_N, Ldg_Load_Thresh_Lower=SensorModel.WOW.Cell.loadThresholdLower_N, TO_Persist_Time=SensorModel.WOW.Cell.TO_persistanceTime_s, TO_Latch_Time=SensorModel.WOW.Cell.TO_latchTime_s, TO_Load_Thresh=SensorModel.WOW.Cell.TO_loadThreshold_N, DSCnumBits=24, numBits=16, satMaxMG=15000, satMinMG=-300, dscNoiseMG=1, DSCRangeMaxMG=15000, DSCRangeMinMG=-15000, satMaxNG=1000, satMinNG=-250, dscNoiseNG=0.25, DSCRangeMaxNG=1000, DSCRangeMinNG=-1000, cellSatMaxMG=15000, cellSatMinMG=-15000, cell2WheelFactorMG=5.98, cellSatMaxNG=1000, cellSatMinNG=-1000, cell2WheelFactorNG=1}
      mask prompts: Ldg_Persist_Time "Landing Persistance Time [s]"; Ldg_Latch_Time_P "Primary Landing Latch Time [s]"; Ldg_Latch_Time_S "Secondary Landing Latch Time [s]"; Ldg_Load_Thresh_Upper "Landing Load Threshold Upper [N]"; Ldg_Load_Thresh_Lower "Landing Load Threshold Lower [N]"; TO_Persist_Time "Take Off Persistance Time [s]"; TO_Latch_Time "Take Off Latch Time [s]"; TO_Load_Thresh "Take Off Load Threshold  [N]"; DSCnumBits "DSC Encoded Resolution [num bits]"; numBits "CANBridge Encoded Resolution [num bits]"; satMaxMG "Main Gear CANBridge Saturation Max [N]"; satMinMG "Main Gear CANBridge Saturation Min [N]"; dscNoiseMG "Main Gear DSC Noise Level pk-pk [N]"; DSCRangeMaxMG "Main Gear DSC Range Max [N]"; DSCRangeMinMG "Main Gear DSC Range Min [N]"; satMaxNG "Nose Gear CANBridge Saturation Max [N]"; satMinNG "Nose Gear CANBridge Saturation Min [N]"; dscNoiseNG "Nose Gear DSC Noise Level pk-pk [N]"; DSCRangeMaxNG "Nose Gear DSC Range Max [N]"; DSCRangeMinNG "Nose Gear DSC Range Min [N]"; cellSatMaxMG "Main Gear Cell Saturation Max [N]"; cellSatMinMG "Main Gear Cell Saturation Min [N]"; cell2WheelFactorMG "Main Gear Cell to Wheel Load Scale Factor"; cellSatMaxNG "Nose Gear Cell Saturation Max [N]"; cellSatMinNG "Nose Gear Cell Saturation Min [N]"; cell2WheelFactorNG "Nose Gear Cell to Wheel Load Scale Factor"
      mask DialogControl DescGroupVar Prompt: Full model of load-cell based weight-on-wheels system.
      mask DialogControl LogicGroupVar Prompt: Logic Configuration
      mask DialogControl DataGroupVar Prompt: Data Acquisition
      mask DialogControl Container5 Prompt: MG
      mask DialogControl Container6 Prompt: NG
      mask DialogControl ParamGroupVar Prompt: Physical Parameters
      mask DialogControl Container8 Prompt: MG
      mask DialogControl Container9 Prompt: NG
  Load Cell WoW Model 8 : Subsystem  VariantControl="SensorModel.WOW.Cell.Variant==\"LOAD8\""
  Load Cell WoW Model 9 : Subsystem  VariantControl="SensorModel.WOW.Cell.Variant==\"LOAD9\""
